simulink model "BasicQuadrotorControl"  (R2014b)
settings: Solver=FixedStepDiscrete  StartTime=0.0  StopTime=4000  FixedStep=1  RelTol=1e-3
libraries: hdlsllib x11, simulink x5
settings Model: Creator=bsoheili  LastModifiedBy=dlwalter
settings DataIOCC: SaveOutput=off  SaveTime=off
settings OptimizationCC: BlockReduction=off  ConditionallyExecuteInputs=off  InlineParams=on  UseDivisionForNetSlopeComputation=UseDivisionForReciprocalsOfIntegersOnly  UseFloatMulNetSlope=on  InlineInvariantSignals=on  EnhancedBackFolding=on  EfficientFloat2IntCast=on  OptimizeModelRefInitCode=on  LifeSpan=1
settings DebuggingCC: AlgebraicLoopMsg=error  InheritedTsInSrcMsg=none  StrictBusMsg=ErrorOnBusTreatedAsVector  NonBusSignalsTreatedAsBus=error
settings HardwareCC: ProdHWDeviceType=ASIC/FPGA->ASIC/FPGA  ProdEqTarget=off
settings RTWCC: SystemTargetFile=ert.tlc  TemplateMakefile=ert_default_tmf  Description=Embedded Coder  GenerateReport=on  ProcessScript=ert_make_rtw_hook  IncludeHyperlinkInReport=on  LaunchReport=on  GenerateTraceInfo=on  GenerateTraceReport=on  GenerateTraceReportSl=on  GenerateTraceReportSf=on  GenerateTraceReportEml=on  GenerateCodeMetricsReport=on
settings CodeAppCC: IgnoreCustomStorageClasses=off
settings ERTTargetCC: GenerateSampleERTMain=on  CombineSignalStateStructs=on  SuppressErrorStatus=on  InlinedParameterPlacement=NonHierarchical  ERTCustomFileTemplate=example_file_process.tlc

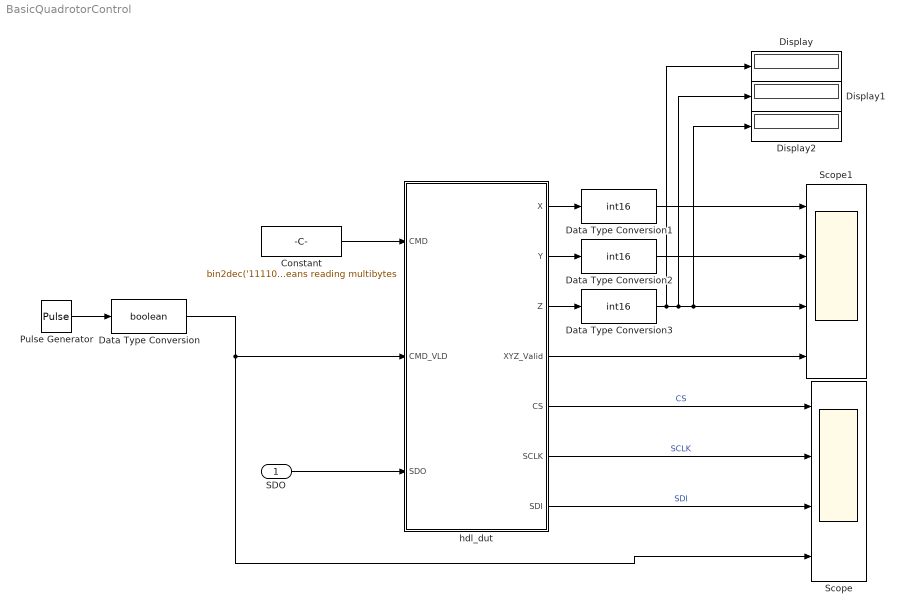
== system BasicQuadrotorControl ==
  SDO : Inport  OutDataTypeStr=boolean
  Constant : Constant  Value="bin2dec('1111001100110011')  % 11 in msb means reading multibytes"  OutDataTypeStr=fixdt(0,16,0)  SampleTime=-1
  Data Type Conversion : DataTypeConversion  OutDataTypeStr=boolean
  Data Type Conversion1 : DataTypeConversion  OutDataTypeStr=int16
  Data Type Conversion2 : DataTypeConversion  OutDataTypeStr=int16
  Data Type Conversion3 : DataTypeConversion  OutDataTypeStr=int16
  Display : Display
  Display1 : Display
  Display2 : Display
  Pulse Generator : DiscretePulseGenerator  Period=500  PhaseDelay=53
  Scope : Scope  NumInputPorts=4
      settings: TickLabels=on  TimeRange=2000  YMin=-5~-5~-5~-5  YMax=5~5~5~5
  Scope1 : Scope  NumInputPorts=4
      settings: TickLabels=on  TimeRange=2000  YMin=-5~-5~-5~-5  YMax=5~5~5~5  SaveName=ScopeData2
  hdl_dut : Subsystem  TreatAsAtomicUnit=on
  wires:
  Data Type Conversion/1 -> Scope/4, hdl_dut/2(CMD_VLD)
  SDO/1 -> hdl_dut/3(SDO)
  hdl_dut/1(X) -> Data Type Conversion1/1
  hdl_dut/2(Y) -> Data Type Conversion2/1
  hdl_dut/3(Z) -> Data Type Conversion3/1
  hdl_dut/5(CS) -> Scope/1  "CS"
  hdl_dut/6(SCLK) -> Scope/2  "SCLK"
  hdl_dut/7(SDI) -> Scope/3  "SDI"
  Pulse Generator/1 -> Data Type Conversion/1
  Constant/1 -> hdl_dut/1(CMD)
  hdl_dut/4(XYZ_Valid) -> Scope1/4
  Data Type Conversion1/1 -> Scope1/1
  Data Type Conversion2/1 -> Scope1/2
  Data Type Conversion3/1 -> Display/1, Display1/1, Display2/1, Scope1/3

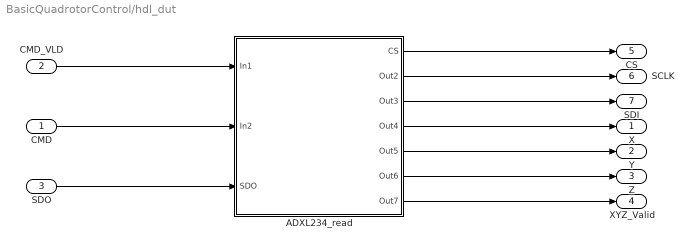
== system BasicQuadrotorControl/hdl_dut ==
  CMD : Inport
  CMD_VLD : Inport  Port=2
  SDO : Inport  Port=3
  ADXL234_read : Subsystem  TreatAsAtomicUnit=on
  X : Outport
  Y : Outport  Port=2
  Z : Outport  Port=3
  XYZ_Valid : Outport  Port=4
  CS : Outport  Port=5
  SCLK : Outport  Port=6
  SDI : Outport  Port=7
  wires:
  CMD_VLD/1 -> ADXL234_read/1(In1)
  CMD/1 -> ADXL234_read/2(In2)
  SDO/1 -> ADXL234_read/3(SDO)
  ADXL234_read/1(CS) -> CS/1
  ADXL234_read/2(Out2) -> SCLK/1
  ADXL234_read/3(Out3) -> SDI/1
  ADXL234_read/4(Out4) -> X/1
  ADXL234_read/5(Out5) -> Y/1
  ADXL234_read/6(Out6) -> Z/1
  ADXL234_read/7(Out7) -> XYZ_Valid/1

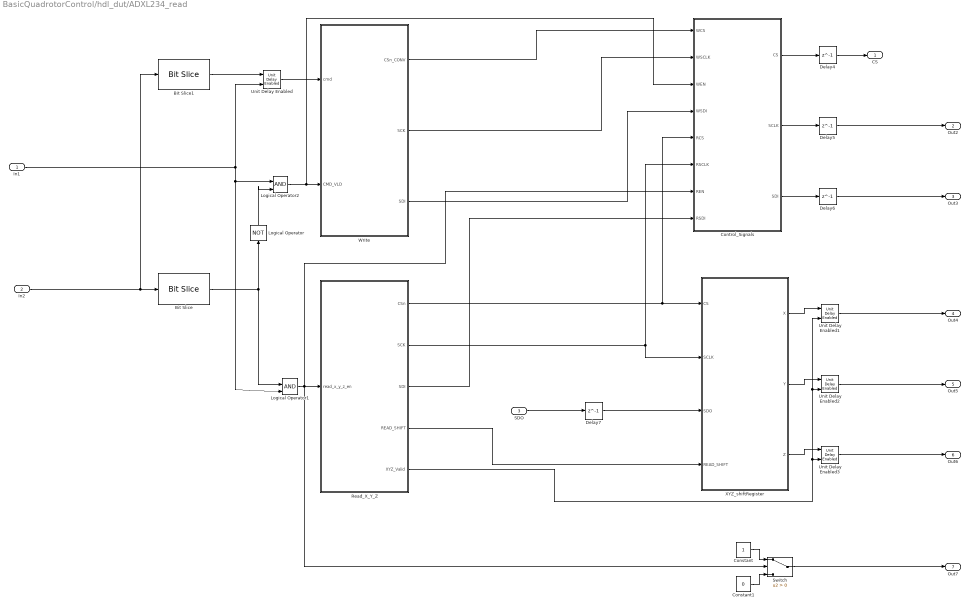
== system BasicQuadrotorControl/hdl_dut/ADXL234_read ==
  In1 : Inport
  In2 : Inport  Port=2
  SDO : Inport  Port=3
  Bit Slice : hdlsllib/HDL Operations/Bit Slice  lidx=15  ridx=15
  Bit Slice1 : hdlsllib/HDL Operations/Bit Slice  lidx=13  ridx=0
  Constant : Constant  OutDataTypeStr=boolean
  Constant1 : Constant  Value=0  OutDataTypeStr=boolean
  Control_Signals : Subsystem
  Delay{4..7} (4 alike) : Delay  DelayLength=1  InitialCondition=0
  Logical Operator : Logic  Operator=NOT  IconShape=distinctive  AllPortsSameDT=off  OutDataTypeStr=boolean
  Logical Operator1 : Logic  IconShape=distinctive  AllPortsSameDT=off  OutDataTypeStr=boolean
  Logical Operator2 : Logic  IconShape=distinctive  AllPortsSameDT=off  OutDataTypeStr=boolean
  Read_X_Y_Z : Stateflow chart  TreatAsAtomicUnit=on
  Switch : Switch  Criteria=u2 > Threshold
  Unit Delay Enabled{,1..3} (4 alike) : simulink/Additional Math & Discrete/Additional Discrete/Unit Delay Enabled  vinit=0.0  tsamp=-1
  Write : Stateflow chart  TreatAsAtomicUnit=on
  XYZ_shiftRegister : Subsystem
  CS : Outport
  Out2 : Outport  Port=2
  Out3 : Outport  Port=3
  Out4 : Outport  Port=4
  Out5 : Outport  Port=5
  Out6 : Outport  Port=6
  Out7 : Outport  Port=7
  wires:
  In2/1 -> Bit Slice1/1, Bit Slice/1
  Bit Slice/1 -> Logical Operator/1, Logical Operator1/1
  Logical Operator1/1 -> Switch/2, Control_Signals/7(REN), Read_X_Y_Z/1(read_x_y_z_en)
  In1/1 -> Unit Delay Enabled/2, Logical Operator1/2, Logical Operator2/1
  Write/1(CSn_CONV) -> Control_Signals/1(WCS)
  Delay4/1 -> CS/1
  Constant/1 -> Switch/1
  SDO/1 -> Delay7/1
  Delay7/1 -> XYZ_shiftRegister/3(SDO)
  Write/2(SCK) -> Control_Signals/2(WSCLK)
  Control_Signals/3(SDI) -> Delay6/1
  XYZ_shiftRegister/1(X) -> Unit Delay Enabled1/1
  Control_Signals/2(SCLK) -> Delay5/1
  Logical Operator2/1 -> Control_Signals/3(WEN), Write/2(CMD_VLD)
  Write/3(SDI) -> Control_Signals/4(WSDI)
  Unit Delay Enabled3/1 -> Out6/1
  Control_Signals/1(CS) -> Delay4/1
  Unit Delay Enabled/1 -> Write/1(cmd)
  Logical Operator/1 -> Logical Operator2/2
  Read_X_Y_Z/3(SDI) -> Control_Signals/8(RSDI)
  XYZ_shiftRegister/2(Y) -> Unit Delay Enabled2/1
  Delay6/1 -> Out3/1
  Constant1/1 -> Switch/3
  XYZ_shiftRegister/3(Z) -> Unit Delay Enabled3/1
  Bit Slice1/1 -> Unit Delay Enabled/1
  Read_X_Y_Z/5(XYZ_Valid) -> Unit Delay Enabled3/2, Unit Delay Enabled2/2, Unit Delay Enabled1/2
  Read_X_Y_Z/1(CSn) -> Control_Signals/5(RCS), XYZ_shiftRegister/1(CS)
  Delay5/1 -> Out2/1
  Read_X_Y_Z/2(SCK) -> Control_Signals/6(RSCLK), XYZ_shiftRegister/2(SCLK)
  Unit Delay Enabled2/1 -> Out5/1
  Read_X_Y_Z/4(READ_SHIFT) -> XYZ_shiftRegister/4(READ_SHIFT)
  Switch/1 -> Out7/1
  Unit Delay Enabled1/1 -> Out4/1

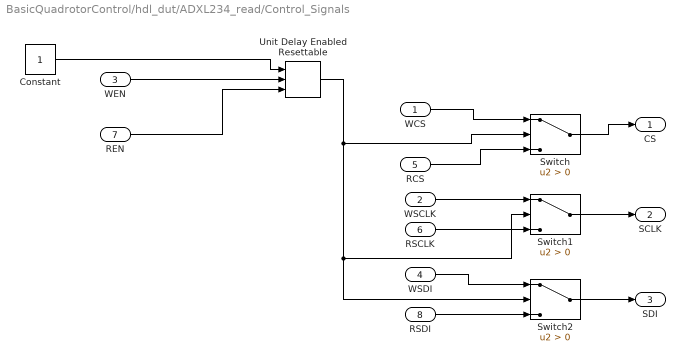
== system BasicQuadrotorControl/hdl_dut/ADXL234_read/Control_Signals ==
  WCS : Inport
  WSCLK : Inport  Port=2
  WEN : Inport  Port=3
  WSDI : Inport  Port=4
  RCS : Inport  Port=5
  RSCLK : Inport  Port=6
  REN : Inport  Port=7
  RSDI : Inport  Port=8
  Constant : Constant  OutDataTypeStr=boolean  SampleTime=-1
  Switch : Switch  Criteria=u2 > Threshold
  Switch1 : Switch  Criteria=u2 > Threshold
  Switch2 : Switch  Criteria=u2 > Threshold
  Unit Delay Enabled Resettable : simulink/Additional Math & Discrete/Additional Discrete/Unit Delay Enabled Resettable  vinit=0.0  tsamp=-1
  CS : Outport
  SCLK : Outport  Port=2
  SDI : Outport  Port=3
  wires:
  WCS/1 -> Switch/1
  WSCLK/1 -> Switch1/1
  WSDI/1 -> Switch2/1
  RSDI/1 -> Switch2/3
  Switch2/1 -> SDI/1
  Switch/1 -> CS/1
  Switch1/1 -> SCLK/1
  Unit Delay Enabled Resettable/1 -> Switch/2, Switch1/2, Switch2/2
  Constant/1 -> Unit Delay Enabled Resettable/1
  WEN/1 -> Unit Delay Enabled Resettable/2
  RSCLK/1 -> Switch1/3
  REN/1 -> Unit Delay Enabled Resettable/3
  RCS/1 -> Switch/3

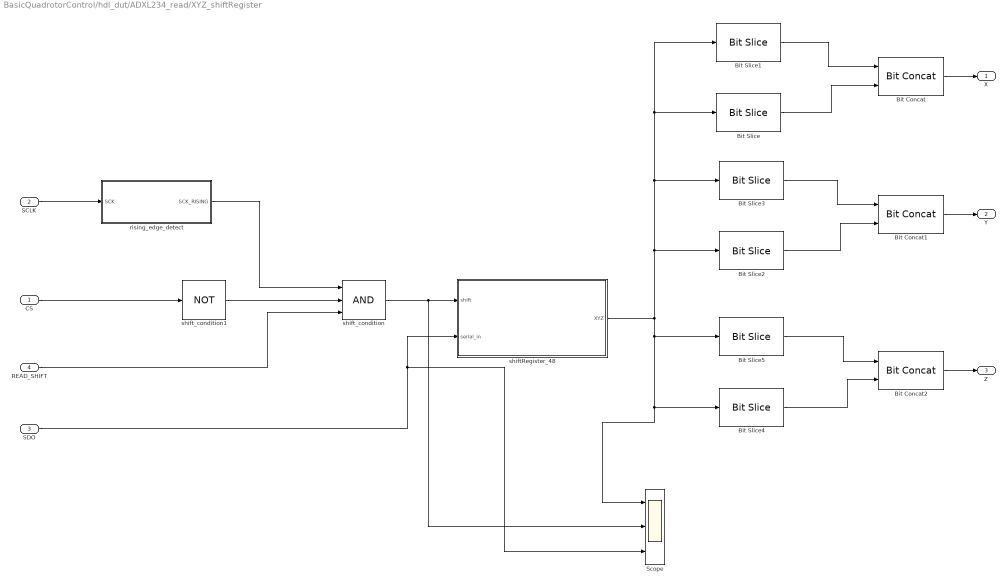
== system BasicQuadrotorControl/hdl_dut/ADXL234_read/XYZ_shiftRegister ==
  CS : Inport
  SCLK : Inport  Port=2
  SDO : Inport  Port=3
  READ_SHIFT : Inport  Port=4
  Bit Concat : hdlsllib/HDL Operations/Bit Concat  numInputs=2
  Bit Concat1 : hdlsllib/HDL Operations/Bit Concat  numInputs=2
  Bit Concat2 : hdlsllib/HDL Operations/Bit Concat  numInputs=2
  Bit Slice : hdlsllib/HDL Operations/Bit Slice  lidx=47  ridx=40
  Bit Slice1 : hdlsllib/HDL Operations/Bit Slice  lidx=39  ridx=32
  Bit Slice2 : hdlsllib/HDL Operations/Bit Slice  lidx=31  ridx=24
  Bit Slice3 : hdlsllib/HDL Operations/Bit Slice  lidx=23  ridx=16
  Bit Slice4 : hdlsllib/HDL Operations/Bit Slice  lidx=15  ridx=8
  Bit Slice5 : hdlsllib/HDL Operations/Bit Slice  lidx=7  ridx=0
  Scope : Scope  NumInputPorts=3
      settings: TickLabels=on  YMin=-5~-5~-5  YMax=5~5~5  SaveName=ScopeData3
  rising_edge_detect : Subsystem  Description=This section detects the rising edge of the SCK input.
  shiftRegister_48 : MATLAB Function  TreatAsAtomicUnit=on
  shift_condition : Logic  Inputs=3  IconShape=distinctive  AllPortsSameDT=off  OutDataTypeStr=boolean
  shift_condition1 : Logic  Operator=NOT  Inputs=3  IconShape=distinctive  AllPortsSameDT=off  OutDataTypeStr=boolean
  X : Outport
  Y : Outport  Port=2
  Z : Outport  Port=3
  wires:
  SCLK/1 -> rising_edge_detect/1(SCK)
  rising_edge_detect/1(SCK_RISING) -> shift_condition/1
  CS/1 -> shift_condition1/1
  shift_condition1/1 -> shift_condition/2
  READ_SHIFT/1 -> shift_condition/3
  shift_condition/1 -> Scope/2, shiftRegister_48/1(shift)
  SDO/1 -> Scope/3, shiftRegister_48/2(serial_in)
  Bit Slice1/1 -> Bit Concat/1
  Bit Slice/1 -> Bit Concat/2
  Bit Concat/1 -> X/1
  shiftRegister_48/1(XYZ) -> Bit Slice2/1, Bit Slice3/1, Bit Slice/1, Bit Slice1/1, Bit Slice5/1, Bit Slice4/1, Scope/1
  Bit Slice3/1 -> Bit Concat1/1
  Bit Slice2/1 -> Bit Concat1/2
  Bit Concat1/1 -> Y/1
  Bit Slice5/1 -> Bit Concat2/1
  Bit Slice4/1 -> Bit Concat2/2
  Bit Concat2/1 -> Z/1

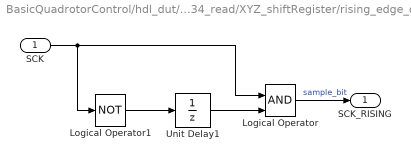
== system BasicQuadrotorControl/hdl_dut/ADXL234_read/XYZ_shiftRegister/rising_edge_detect ==
  SCK : Inport
  Logical Operator : Logic  IconShape=distinctive  AllPortsSameDT=off  OutDataTypeStr=boolean
  Logical Operator1 : Logic  Operator=NOT  IconShape=distinctive  AllPortsSameDT=off  OutDataTypeStr=boolean
  Unit Delay1 : UnitDelay  SampleTime=-1
  SCK_RISING : Outport
  wires:
  Logical Operator1/1 -> Unit Delay1/1
  Unit Delay1/1 -> Logical Operator/2
  Logical Operator/1 -> SCK_RISING/1  "sample_bit"
  SCK/1 -> Logical Operator/1, Logical Operator1/1

== matlab function BasicQuadrotorControl/hdl_dut/ADXL234_read/XYZ_shiftRegister/shiftRegister_48 ==
  data: shift input boolean; serial_in input; XYZ output fixdt(0,48,0)
function XYZ = fcn(shift, serial_in)
%#codegen

%%
persistent XYZ_int 
if isempty(XYZ_int)
    XYZ_int = fi(0,0,48,0);
end
%%


%%
if shift == true 
    serial_in_int = fi(serial_in, 0, 1, 0);
    XYZ_int = bitsll(XYZ_int, 1);
    XYZ_int = (bitconcat(bitsliceget(XYZ_int, 48, 2), serial_in_int));
end
%%
XYZ = XYZ_int;
%%

== stateflow chart BasicQuadrotorControl/hdl_dut/ADXL234_read/Write ==
  settings: executeAtInitialization=1
  note: This is single write to and address location. The write and MB bist
      | are hard coded. The 'cmd' is 14 bits. The upper 6 bits are address and
      | the lower 8 bits are data.
      | Here is the address map :
  state IDLE
  note: ?
  state START_CONV
    settings: description=|
        | During START_CONV the CSn_CONV is held high for 10 clock cycles.
        | Assuming the FPGA clock frequency is 100 MHz, the 10 clock count delay
        | provides 100 nS delay which is the typical time specified in the ADC data
        | sheet for the CSn_CONV input to the ADC.
        | 
        | The count comparator can be changed from 10 by the user as long as the ADC requirment for minimum of 40 nS is met.
  state tCONV_delay
    settings: description="tCoONV time is typical 3 uS and Maximum 3.5 uS according to ADC data sheet.  Assuming clock frequency of 100 MHz, the maximum count value for 3 uS delay should be (3 uS/10 nS=) 300."
  state START_ADC_RDWR
    settings: description="The ADC maximum clock frequency, according to ADC data sheet, is rated at 40 MHz.  Assuming a 100 MHz FPGA clock dividing the FPGA clock by 3 to generate a 33.33 MHz ADC clock (SCK) for the ADC."
  state CLOCKING
    settings: description="tCoONV time is typical 3 uS and Maximum 3.5 uS according to ADC data sheet.  Assuming clock frequency of 100 MHz, the maximum count value for 3 uS delay should be (3 uS/10 nS=) 300."
  state END1
  state END
  (default) -> IDLE
  END -> IDLE
  IDLE -> START_CONV : [CMD_VLD == true]{CSn_CONV = false;...
      | SCK = false;
      | SDI = false; } % sdi_gen(cmd ,clock_cnt);}
  START_CONV -> START_CONV [order 2] : {count++;}
  START_CONV -> tCONV_delay [order 1] : [count == 10]{count = 0; CSn_CONV = false; SCK = true;}
  tCONV_delay -> tCONV_delay [order 2] : {count++;}
  tCONV_delay -> START_ADC_RDWR [order 1] : [count ==10]...
      | {count = 0;
      | SCK = false;}
  CLOCKING -> CLOCKING [order 2] : {count++;}
  START_ADC_RDWR -> START_ADC_RDWR [order 3] : {count++;}
  START_ADC_RDWR -> CLOCKING [order 2] : [count == 10]{count = 0;SCK=true;clock_cnt++;}
  CLOCKING -> START_ADC_RDWR [order 1] : [count == 10]{count = 0;...
      | SCK=false;
      | SDI = sdi_gen(cmd,clock_cnt);}
  START_ADC_RDWR -> END1 [order 1] : [clock_cnt == 14  && count == 10]...
      | {clock_cnt = 0;...
      | count = 0;
      | SCK = true;}
  END1 -> END1 [order 2] : {count++;}
  END1 -> END [order 1] : [count == 10]{count = 0; CSn_CONV = true;}
  data: word function_input fixdt(0,14,0); cnt function_input fixdt(0,5,0); ser_data function_output boolean; CSn_CONV output boolean =true; count local fixdt(0,9,0) =0; SCK output boolean =true; clock_cnt local fixdt(0,5,0) =0; SDI output boolean =true; cmd input fixdt(0,14,0); CMD_VLD input boolean
  function ser_data = sdi_gen(word,cnt):
    | function ser_data = sdi_gen(word,cnt)
    | 
    | 
    | persistent ser_data_int;
    | if isempty(ser_data_int)
    |     ser_data_int = false;
    | end
    | 
    | 
    | if cnt == fi(1,0,5,0)
    |     ser_data_int = logical(bitget(word, 14));
    | elseif cnt == fi(2,0,5,0)
    |     ser_data_int = logical(bitget(word, 13));
    | elseif cnt == fi(3,0,5,0)
    |     ser_data_int = logical(bitget(word, 12));
    | elseif cnt == fi(4,0,5,0)
    |     ser_data_int = logical(bitget(word, 11));
    | elseif cnt == fi(5,0,5,0)
    |     ser_data_int = logical(bitget(word, 10));
    | elseif cnt == fi(6,0,5,0)
    |     ser_data_int = logical(bitget(word, 9));
    | elseif cnt == fi(7,0,5,0)
    |     ser_data_int = logical(bitget(word, 8));
    | elseif cnt == fi(8,0,5,0)
    |     ser_data_int = logical(bitget(word, 7));
    | elseif cnt == fi(9,0,5,0)
    |     ser_data_int = logical(bitget(word, 6));
    | elseif cnt == fi(10,0,5,0)
    |     ser_data_int = logical(bitget(word, 5));
    | elseif cnt == fi(11,0,5,0)
    |     ser_data_int = logical(bitget(word, 4));
    | elseif cnt == fi(12,0,5,0)
    |     ser_data_int = logical(bitget(word, 3));
    | elseif cnt == fi(13,0,5,0)
    |     ser_data_int = logical(bitget(word, 2));
    | elseif cnt == fi(14,0,5,0)
    |     ser_data_int = logical(bitget(word, 1));
    | else
    |     ser_data_int = false;
    | end
    | 
    | ser_data = ser_data_int;

== stateflow chart BasicQuadrotorControl/hdl_dut/ADXL234_read/Read_X_Y_Z ==
  settings: executeAtInitialization=1
  state IDLE
  note: This chart reads the six X, Y, Z registers from ADXL345 chip
      |
      | !!!!!! Under construction !!!!!!
  note: ?
  state START_CONV
    settings: description=|
        | During START_CONV the CSn_CONV is held high for 10 clock cycles.
        | Assuming the FPGA clock frequency is 100 MHz, the 10 clock count delay
        | provides 100 nS delay which is the typical time specified in the ADC data
        | sheet for the CSn_CONV input to the ADC.
        | 
        | The count comparator can be changed from 10 by the user as long as the ADC requirment for minimum of 40 nS is met.
  state tCONV_delay
    settings: description="tCoONV time is typical 3 uS and Maximum 3.5 uS according to ADC data sheet.  Assuming clock frequency of 100 MHz, the maximum count value for 3 uS delay should be (3 uS/10 nS=) 300."
  state START_ADC_RDWR
    settings: description="The ADC maximum clock frequency, according to ADC data sheet, is rated at 40 MHz.  Assuming a 100 MHz FPGA clock dividing the FPGA clock by 3 to generate a 33.33 MHz ADC clock (SCK) for the ADC."
  state CLOCKING
    settings: description="tCoONV time is typical 3 uS and Maximum 3.5 uS according to ADC data sheet.  Assuming clock frequency of 100 MHz, the maximum count value for 3 uS delay should be (3 uS/10 nS=) 300."
  state Read1
  state Read
  state END
  END -> IDLE [order 1] : [count == 10]...
      | {CSn = true;
      | count = 0;
      | XYZ_Valid = true;
      | READ_SHIFT = false;}
  (default) -> IDLE
  IDLE -> START_CONV : [read_x_y_z_en == true]{CSn = false;
      | clock_cnt++;
      | XYZ_Valid = false;}
  START_CONV -> START_CONV [order 2] : {count++;}
  START_CONV -> tCONV_delay [order 1] : [count == 10]{count = 0; SCK = false;
      |   SDI = sdi_gen(cmd, clock_cnt);} % sending Read bit
  tCONV_delay -> tCONV_delay [order 2] : {count++;}
  tCONV_delay -> START_ADC_RDWR [order 1] : [count ==10]...
      | {count = 0;
      | SCK = true;
      | clock_cnt++;}
  CLOCKING -> CLOCKING [order 2] : {count++;}
  START_ADC_RDWR -> START_ADC_RDWR [order 3] : {count++;}
  START_ADC_RDWR -> CLOCKING [order 2] : [count == 10]{count = 0;SCK= false; SDI = sdi_gen(cmd, clock_cnt);}
  CLOCKING -> START_ADC_RDWR [order 1] : [count == 10]{count = 0;...
      | SCK=true;
      | clock_cnt++;}
  START_ADC_RDWR -> Read [order 1] : [clock_cnt == 9  && count == 10]...
      | {count = 0;
      | SCK = false;
      | SDI = true;
      | READ_SHIFT = true;}
  Read1 -> Read1 [order 2] : {count++;}
  Read -> Read1 [order 2] : [count == 10]{SCK = true;count = 0; clock_cnt++;}
  Read -> Read [order 3] : {count++;}
  Read1 -> Read [order 1] : [count == 10]{SCK = false;count = 0;}
  Read -> END [order 1] : [count == 10 && clock_cnt == 56]...
      | {count = 0;
      | clock_cnt = 0;
      | SCK = true;}
  END -> END [order 2] : {count++;}
  data: word function_input uint8; cnt function_input fixdt(0,5,0); ser_data function_output boolean; read_x_y_z_en input boolean; CSn output boolean =true; count local fixdt(0,9,0) =0; SCK output boolean =true; clock_cnt local fixdt(0,6,0) =0; SDI output boolean =true; cmd constant uint8 =242; READ_SHIFT output boolean =false; XYZ_Valid output boolean =true
  function ser_data = sdi_gen(word,cnt):
    | function ser_data = sdi_gen(word,cnt)
    | 
    | 
    | persistent ser_data_int;
    | if isempty(ser_data_int)
    |     ser_data_int = false;
    | end
    | 
    | 
    | if cnt == fi(1,0,5,0)
    |     ser_data_int = logical(bitget(word, 8));
    | elseif cnt == fi(2,0,5,0)
    |     ser_data_int = logical(bitget(word, 7));
    | elseif cnt == fi(3,0,5,0)
    |     ser_data_int = logical(bitget(word, 6));
    | elseif cnt == fi(4,0,5,0)
    |     ser_data_int = logical(bitget(word, 5));
    | elseif cnt == fi(5,0,5,0)
    |     ser_data_int = logical(bitget(word, 4));
    | elseif cnt == fi(6,0,5,0)
    |     ser_data_int = logical(bitget(word, 3));
    | elseif cnt == fi(7,0,5,0)
    |     ser_data_int = logical(bitget(word, 2));
    | elseif cnt == fi(8,0,5,0)
    |     ser_data_int = logical(bitget(word, 1));
    | else
    |     ser_data_int = true;
    | end
    | 
    | ser_data = ser_data_int;
